simulink model "quadcopter_wind"  (Simulink 9.0)
settings: Solver=ode45  StartTime=0.0  StopTime=30  FixedStep=0.001  RelTol=1e-3  EnableMultiTasking=on
values from neighbouring files (symbols this model uses):
  C = 1    [control_params.m]
  f_phi = 10    [control_params.m]
  f_psi = 0.1    [control_params.m]
  f_theta = 0.1    [control_params.m]
  f_x = 10    [control_params.m]
  f_y = 10    [control_params.m]
  f_z = 10    [control_params.m]
  g = 9.8    [control_params.m]
  J_1 = 1    [control_params.m]
  J_2 = 1    [control_params.m]
  J_3 = 1    [control_params.m]
  l = 0.5    [control_params.m]
  m = 1    [control_params.m]
  phi_desired = 1    [control_params.m]
  x_desired = 1    [control_params.m]
  y_desired = 1    [control_params.m]
  z_desired = 1    [control_params.m]
settings Model: Creator=Oleg Borisov  LastModifiedBy=broth
settings DataIOCC: LimitDataPoints=on  SignalLoggingSaveFormat=ModelDataLogs
settings OptimizationCC: ExpressionDepthLimit=2147483647
settings DebuggingCC: SolverPrmCheckMsg=warning  FcnCallInpInsideContextMsg=warning  StateNameClashWarn=warning
settings GRTTargetCC: GeneratePreprocessorConditionals=Disable all  CombineOutputUpdateFcns=off  GRTInterface=on

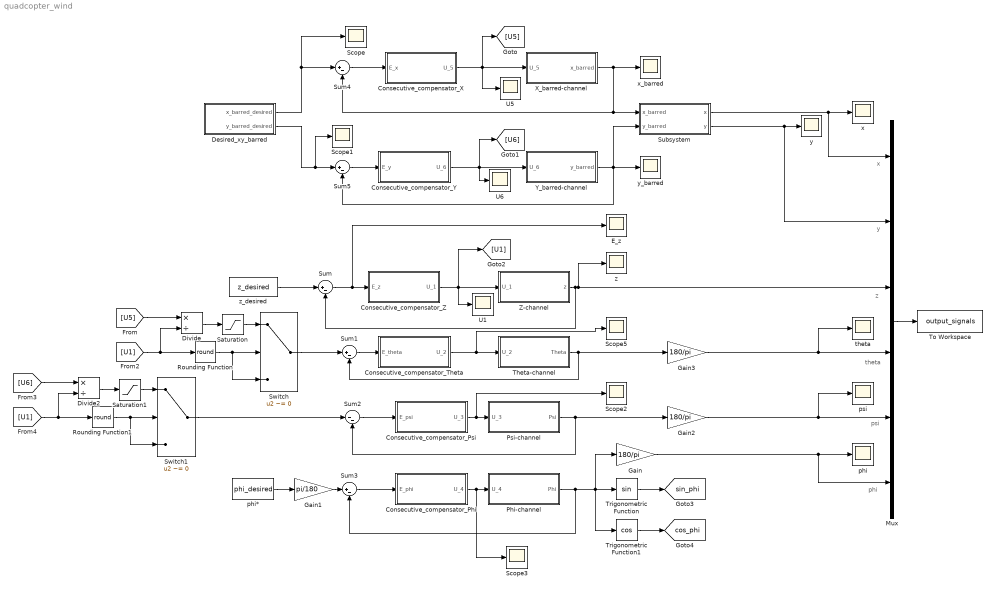
== system quadcopter_wind ==
  note: z
  note: y
  note: x
  note: theta
  note: psi
  note: phi
  Consecutive_compensator_Phi : Subsystem
  Consecutive_compensator_Psi : Subsystem
  Consecutive_compensator_Theta : Subsystem
  Consecutive_compensator_X : Subsystem
  Consecutive_compensator_Y : Subsystem
  Consecutive_compensator_Z : Subsystem
  Desired_xy_barred : Subsystem
  Divide : Product  Inputs=*/
  Divide2 : Product  Inputs=*/
  E_z : Scope
  Gain : Gain  Gain=180/pi
  Gain1 : Gain  Gain=pi/180
  Gain2 : Gain  Gain=180/pi
  Gain3 : Gain  Gain=180/pi
  Mux : Mux  Inputs=6
  Phi-channel : Subsystem
  Psi-channel : Subsystem
  Rounding Function : Rounding  Operator=round
  Rounding Function1 : Rounding  Operator=round
  Saturation : Saturate  UpperLimit=pi/6  LowerLimit=-pi/6
  Saturation1 : Saturate  UpperLimit=pi/6  LowerLimit=-pi/6
  Scope{,1..3,5} (5 alike) : Scope
  Subsystem : Subsystem
  Sum{,1,3..5} (5 alike) : Sum  Inputs=|+-
  Sum2 : Sum  Inputs=|--
  Switch : Switch  Criteria=u2 ~= 0
  Switch1 : Switch  Criteria=u2 ~= 0
  Theta-channel : Subsystem
  To Workspace : ToWorkspace  VariableName=output_signals  SaveFormat=Structure With Time  SampleTime=-1
  Trigonometric Function : Trigonometry
  Trigonometric Function1 : Trigonometry  Operator=cos
  U1 : Scope
  U5 : Scope
  U6 : Scope
  X_barred-channel : Subsystem
  Y_barred-channel : Subsystem
  Z-channel : Subsystem
  phi : Scope
  phi* : Constant  Value=phi_desired
  psi : Scope
  theta : Scope
  x : Scope
  x_barred : Scope
  y : Scope
  y_barred : Scope
  z : Scope
  z_desired : Constant  Value=z_desired
  tag scope: cos_phi=global, sin_phi=global
  wires:
  Z-channel/1(z) -> Mux/3, z/1, Sum/2
  Sum/1 -> E_z/1, Consecutive_compensator_Z/1(E_z)
  Consecutive_compensator_Psi/1(U_3) -> Psi-channel/1(U_3), Scope2/1
  Consecutive_compensator_Phi/1(U_4) -> Phi-channel/1(U_4), Scope3/1
  Theta-channel/1(Theta) -> Sum1/2, Gain3/1
  Sum1/1 -> Consecutive_compensator_Theta/1(E_theta)
  Sum2/1 -> Consecutive_compensator_Psi/1(E_psi)
  Psi-channel/1(Psi) -> Sum2/2, Gain2/1
  Sum3/1 -> Consecutive_compensator_Phi/1(E_phi)
  Phi-channel/1(Phi) -> Sum3/2, Trigonometric Function/1, Trigonometric Function1/1, Gain/1
  Consecutive_compensator_Y/1(U_6) -> Y_barred-channel/1(U_6), [U6], U6/1
  [U5] -> Divide/1
  X_barred-channel/1(x_barred) -> x_barred/1, Subsystem/1(x_barred), Sum4/2
  Sum5/1 -> Consecutive_compensator_Y/1(E_y)
  Y_barred-channel/1(y_barred) -> y_barred/1, Sum5/2, Subsystem/2(y_barred)
  Desired_xy_barred/1(x_barred_desired) -> Sum4/1, Scope/1
  Desired_xy_barred/2(y_barred_desired) -> Sum5/1, Scope1/1
  Trigonometric Function/1 -> [sin_phi]
  Trigonometric Function1/1 -> [cos_phi]
  Gain/1 -> Mux/6, phi/1
  phi*/1 -> Gain1/1
  Gain1/1 -> Sum3/1
  Mux/1 -> To Workspace/1
  Subsystem/1(x) -> Mux/1, x/1
  Subsystem/2(y) -> Mux/2, y/1
  Gain2/1 -> Mux/5, psi/1
  Gain3/1 -> Mux/4, theta/1
  Sum4/1 -> Consecutive_compensator_X/1(E_x)
  Consecutive_compensator_X/1(U_5) -> X_barred-channel/1(U_5), [U5], U5/1
  Consecutive_compensator_Z/1(U_1) -> Z-channel/1(U_1), [U1], U1/1
  z_desired/1 -> Sum/1
  Divide/1 -> Saturation/1
  [U1] -> Divide/2, Rounding Function/1
  Switch/1 -> Sum1/1
  Saturation/1 -> Switch/1
  Rounding Function/1 -> Switch/2, Switch/3
  Consecutive_compensator_Theta/1(U_2) -> Theta-channel/1(U_2), Scope5/1
  [U6] -> Divide2/1
  Divide2/1 -> Saturation1/1
  [U1] -> Divide2/2, Rounding Function1/1
  Saturation1/1 -> Switch1/1
  Rounding Function1/1 -> Switch1/2, Switch1/3
  Switch1/1 -> Sum2/1

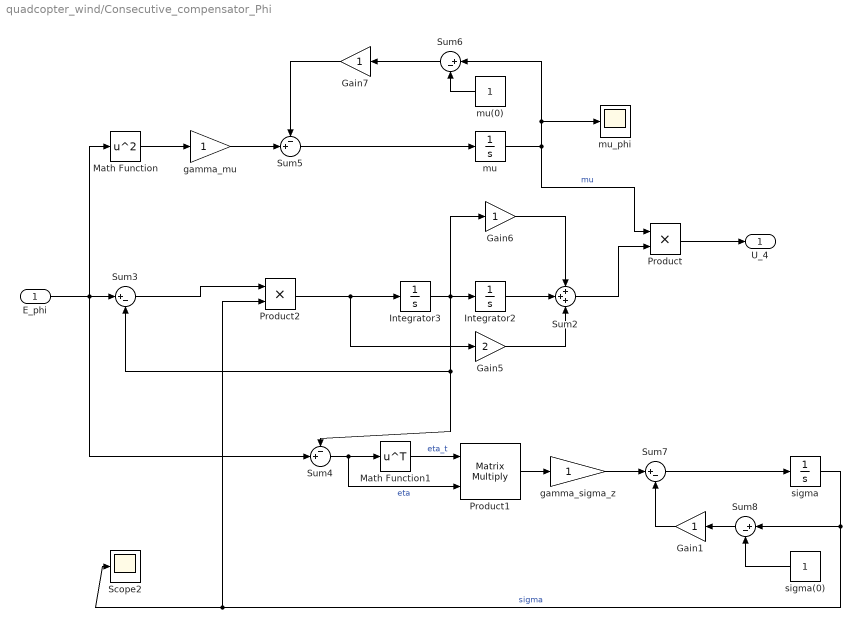
== system quadcopter_wind/Consecutive_compensator_Phi ==
  E_phi : Inport
  Gain1 : Gain
  Gain5 : Gain  Gain=2
  Gain6 : Gain
  Gain7 : Gain
  Integrator2 : Integrator
  Integrator3 : Integrator
  Math Function : Math  Operator=square  SaturateOnIntegerOverflow=on
  Math Function1 : Math  Operator=transpose  SaturateOnIntegerOverflow=on
  Product : Product
  Product1 : Product  Multiplication=Matrix(*)
  Product2 : Product
  Scope2 : Scope
  Sum2 : Sum  Inputs=+++
  Sum{3,6..8} (4 alike) : Sum  Inputs=|+-
  Sum4 : Sum  Inputs=-+|
  Sum5 : Sum  Inputs=-+|
  gamma_mu : Gain
  gamma_sigma_z : Gain
  mu : Integrator  InitialCondition=1
  mu(0) : Constant
  mu_phi : Scope
  sigma : Integrator  InitialCondition=1
  sigma(0) : Constant
  U_4 : Outport
  wires:
  Product2/1 -> Integrator3/1, Gain5/1
  Sum3/1 -> Product2/1
  Integrator2/1 -> Sum2/2
  Product/1 -> U_4/1
  Gain7/1 -> Sum5/1
  Sum2/1 -> Product/2
  mu/1 -> Product/1, mu_phi/1, Sum6/1  "mu"
  Gain6/1 -> Sum2/1
  mu(0)/1 -> Sum6/2
  Gain5/1 -> Sum2/3
  Sum5/1 -> mu/1
  Sum6/1 -> Gain7/1
  gamma_mu/1 -> Sum5/2
  Math Function/1 -> gamma_mu/1
  E_phi/1 -> Sum4/2, Math Function/1, Sum3/1
  Gain1/1 -> Sum7/2
  gamma_sigma_z/1 -> Sum7/1
  Sum7/1 -> sigma/1
  Sum8/1 -> Gain1/1
  sigma(0)/1 -> Sum8/2
  Sum4/1 -> Product1/2, Math Function1/1  "eta"
  Product1/1 -> gamma_sigma_z/1
  Integrator3/1 -> Integrator2/1, Gain6/1, Sum3/2, Sum4/1
  sigma/1 -> Sum8/1, Product2/2, Scope2/1  "sigma"
  Math Function1/1 -> Product1/1  "eta_t"

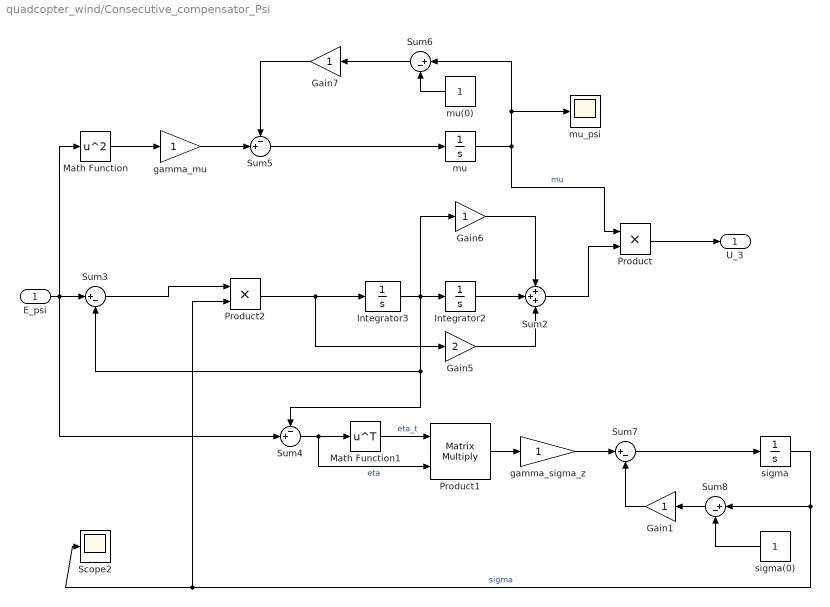
== system quadcopter_wind/Consecutive_compensator_Psi ==
  E_psi : Inport
  Gain1 : Gain
  Gain5 : Gain  Gain=2
  Gain6 : Gain
  Gain7 : Gain
  Integrator2 : Integrator
  Integrator3 : Integrator
  Math Function : Math  Operator=square  SaturateOnIntegerOverflow=on
  Math Function1 : Math  Operator=transpose  SaturateOnIntegerOverflow=on
  Product : Product
  Product1 : Product  Multiplication=Matrix(*)
  Product2 : Product
  Scope2 : Scope
  Sum2 : Sum  Inputs=+++
  Sum{3,6..8} (4 alike) : Sum  Inputs=|+-
  Sum4 : Sum  Inputs=-+|
  Sum5 : Sum  Inputs=-+|
  gamma_mu : Gain
  gamma_sigma_z : Gain
  mu : Integrator  InitialCondition=1
  mu(0) : Constant
  mu_psi : Scope
  sigma : Integrator  InitialCondition=1
  sigma(0) : Constant
  U_3 : Outport
  wires:
  Product2/1 -> Integrator3/1, Gain5/1
  Sum3/1 -> Product2/1
  Integrator2/1 -> Sum2/2
  Product/1 -> U_3/1
  Gain7/1 -> Sum5/1
  Sum2/1 -> Product/2
  mu/1 -> Product/1, mu_psi/1, Sum6/1  "mu"
  Gain6/1 -> Sum2/1
  mu(0)/1 -> Sum6/2
  Gain5/1 -> Sum2/3
  Sum5/1 -> mu/1
  Sum6/1 -> Gain7/1
  gamma_mu/1 -> Sum5/2
  Math Function/1 -> gamma_mu/1
  E_psi/1 -> Math Function/1, Sum4/2, Sum3/1
  Gain1/1 -> Sum7/2
  gamma_sigma_z/1 -> Sum7/1
  Sum7/1 -> sigma/1
  Sum8/1 -> Gain1/1
  sigma(0)/1 -> Sum8/2
  Sum4/1 -> Product1/2, Math Function1/1  "eta"
  Product1/1 -> gamma_sigma_z/1
  Integrator3/1 -> Integrator2/1, Gain6/1, Sum4/1, Sum3/2
  sigma/1 -> Sum8/1, Product2/2, Scope2/1  "sigma"
  Math Function1/1 -> Product1/1  "eta_t"

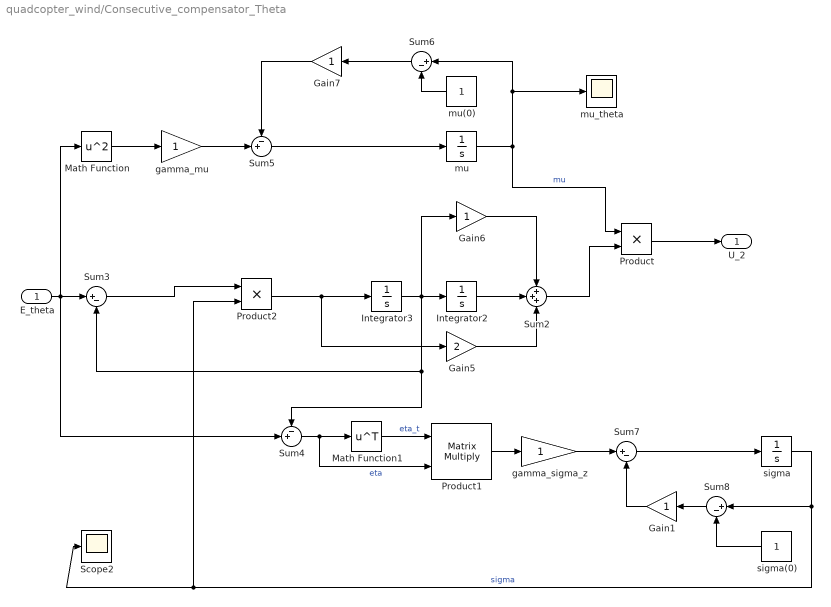
== system quadcopter_wind/Consecutive_compensator_Theta ==
  E_theta : Inport
  Gain1 : Gain
  Gain5 : Gain  Gain=2
  Gain6 : Gain
  Gain7 : Gain
  Integrator2 : Integrator
  Integrator3 : Integrator
  Math Function : Math  Operator=square  SaturateOnIntegerOverflow=on
  Math Function1 : Math  Operator=transpose  SaturateOnIntegerOverflow=on
  Product : Product
  Product1 : Product  Multiplication=Matrix(*)
  Product2 : Product
  Scope2 : Scope
  Sum2 : Sum  Inputs=+++
  Sum{3,6..8} (4 alike) : Sum  Inputs=|+-
  Sum4 : Sum  Inputs=-+|
  Sum5 : Sum  Inputs=-+|
  gamma_mu : Gain
  gamma_sigma_z : Gain
  mu : Integrator  InitialCondition=1
  mu(0) : Constant
  mu_theta : Scope
  sigma : Integrator  InitialCondition=1
  sigma(0) : Constant
  U_2 : Outport
  wires:
  Product2/1 -> Integrator3/1, Gain5/1
  Sum3/1 -> Product2/1
  Integrator2/1 -> Sum2/2
  Product/1 -> U_2/1
  Gain7/1 -> Sum5/1
  Sum2/1 -> Product/2
  mu/1 -> Product/1, mu_theta/1, Sum6/1  "mu"
  Gain6/1 -> Sum2/1
  mu(0)/1 -> Sum6/2
  Gain5/1 -> Sum2/3
  Sum5/1 -> mu/1
  Sum6/1 -> Gain7/1
  gamma_mu/1 -> Sum5/2
  Math Function/1 -> gamma_mu/1
  E_theta/1 -> Sum4/2, Math Function/1, Sum3/1
  Gain1/1 -> Sum7/2
  gamma_sigma_z/1 -> Sum7/1
  Sum7/1 -> sigma/1
  Sum8/1 -> Gain1/1
  sigma(0)/1 -> Sum8/2
  Sum4/1 -> Product1/2, Math Function1/1  "eta"
  Product1/1 -> gamma_sigma_z/1
  Integrator3/1 -> Integrator2/1, Gain6/1, Sum3/2, Sum4/1
  sigma/1 -> Sum8/1, Product2/2, Scope2/1  "sigma"
  Math Function1/1 -> Product1/1  "eta_t"

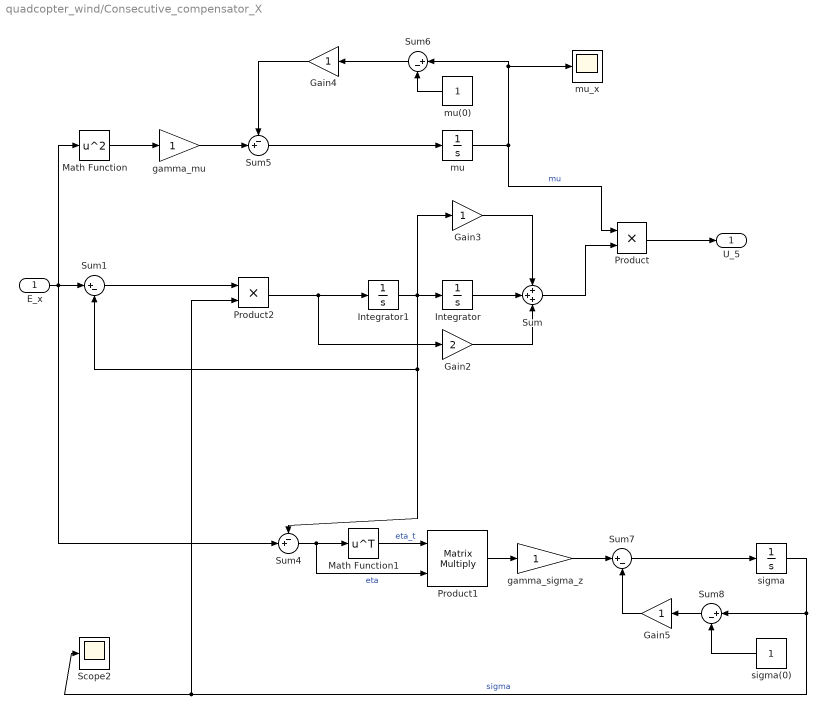
== system quadcopter_wind/Consecutive_compensator_X ==
  E_x : Inport
  Gain2 : Gain  Gain=2
  Gain3 : Gain
  Gain4 : Gain
  Gain5 : Gain
  Integrator : Integrator
  Integrator1 : Integrator
  Math Function : Math  Operator=square  SaturateOnIntegerOverflow=on
  Math Function1 : Math  Operator=transpose  SaturateOnIntegerOverflow=on
  Product : Product
  Product1 : Product  Multiplication=Matrix(*)
  Product2 : Product
  Scope2 : Scope
  Sum : Sum  Inputs=+++
  Sum{1,6..8} (4 alike) : Sum  Inputs=|+-
  Sum4 : Sum  Inputs=-+|
  Sum5 : Sum  Inputs=-+|
  gamma_mu : Gain
  gamma_sigma_z : Gain
  mu : Integrator  InitialCondition=1
  mu(0) : Constant
  mu_x : Scope
  sigma : Integrator  InitialCondition=1
  sigma(0) : Constant
  U_5 : Outport
  wires:
  Sum/1 -> Product/2
  Integrator/1 -> Sum/2
  Sum1/1 -> Product2/1
  Product2/1 -> Integrator1/1, Gain2/1
  Gain3/1 -> Sum/1
  Gain2/1 -> Sum/3
  gamma_mu/1 -> Sum5/2
  mu(0)/1 -> Sum6/2
  Sum6/1 -> Gain4/1
  Math Function/1 -> gamma_mu/1
  mu/1 -> Product/1, mu_x/1, Sum6/1  "mu"
  Gain4/1 -> Sum5/1
  Sum5/1 -> mu/1
  Product/1 -> U_5/1
  sigma(0)/1 -> Sum8/2
  sigma/1 -> Sum8/1, Product2/2, Scope2/1  "sigma"
  Sum8/1 -> Gain5/1
  Math Function1/1 -> Product1/1  "eta_t"
  Gain5/1 -> Sum7/2
  gamma_sigma_z/1 -> Sum7/1
  E_x/1 -> Sum4/2, Math Function/1, Sum1/1
  Integrator1/1 -> Integrator/1, Gain3/1, Sum4/1, Sum1/2
  Sum7/1 -> sigma/1
  Sum4/1 -> Product1/2, Math Function1/1  "eta"
  Product1/1 -> gamma_sigma_z/1

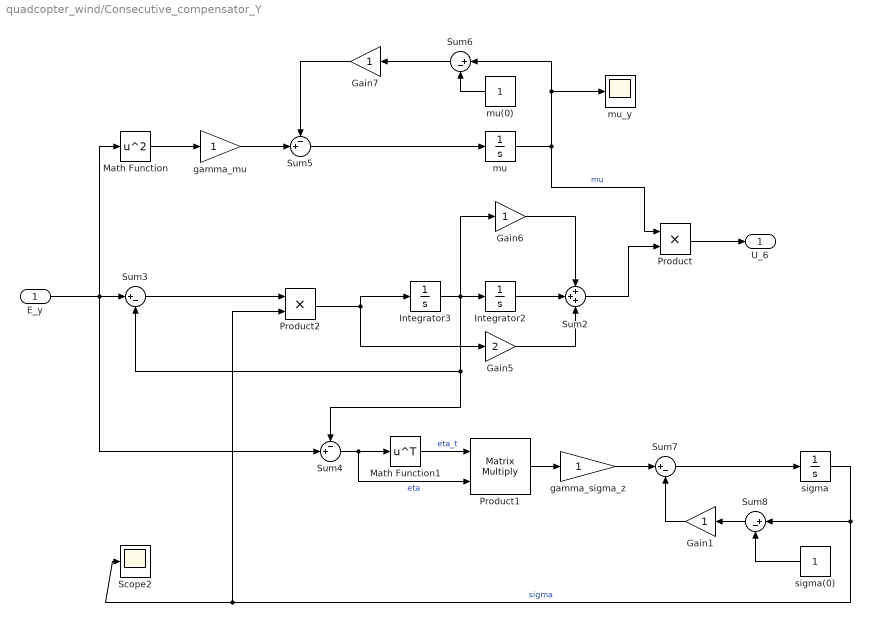
== system quadcopter_wind/Consecutive_compensator_Y ==
  E_y : Inport
  Gain1 : Gain
  Gain5 : Gain  Gain=2
  Gain6 : Gain
  Gain7 : Gain
  Integrator2 : Integrator
  Integrator3 : Integrator
  Math Function : Math  Operator=square  SaturateOnIntegerOverflow=on
  Math Function1 : Math  Operator=transpose  SaturateOnIntegerOverflow=on
  Product : Product
  Product1 : Product  Multiplication=Matrix(*)
  Product2 : Product
  Scope2 : Scope
  Sum2 : Sum  Inputs=+++
  Sum{3,6..8} (4 alike) : Sum  Inputs=|+-
  Sum4 : Sum  Inputs=-+|
  Sum5 : Sum  Inputs=-+|
  gamma_mu : Gain
  gamma_sigma_z : Gain
  mu : Integrator  InitialCondition=1
  mu(0) : Constant
  mu_y : Scope
  sigma : Integrator  InitialCondition=1
  sigma(0) : Constant
  U_6 : Outport
  wires:
  Product/1 -> U_6/1
  Product2/1 -> Integrator3/1, Gain5/1
  Sum3/1 -> Product2/1
  Integrator2/1 -> Sum2/2
  Gain7/1 -> Sum5/1
  Sum2/1 -> Product/2
  mu/1 -> Product/1, mu_y/1, Sum6/1  "mu"
  Gain6/1 -> Sum2/1
  mu(0)/1 -> Sum6/2
  Gain5/1 -> Sum2/3
  Sum5/1 -> mu/1
  Sum6/1 -> Gain7/1
  gamma_mu/1 -> Sum5/2
  Math Function/1 -> gamma_mu/1
  Integrator3/1 -> Integrator2/1, Gain6/1, Sum3/2, Sum4/1
  Sum7/1 -> sigma/1
  gamma_sigma_z/1 -> Sum7/1
  Gain1/1 -> Sum7/2
  Sum4/1 -> Product1/2, Math Function1/1  "eta"
  Sum8/1 -> Gain1/1
  sigma(0)/1 -> Sum8/2
  Product1/1 -> gamma_sigma_z/1
  Math Function1/1 -> Product1/1  "eta_t"
  sigma/1 -> Sum8/1, Product2/2, Scope2/1  "sigma"
  E_y/1 -> Sum3/1, Sum4/2, Math Function/1

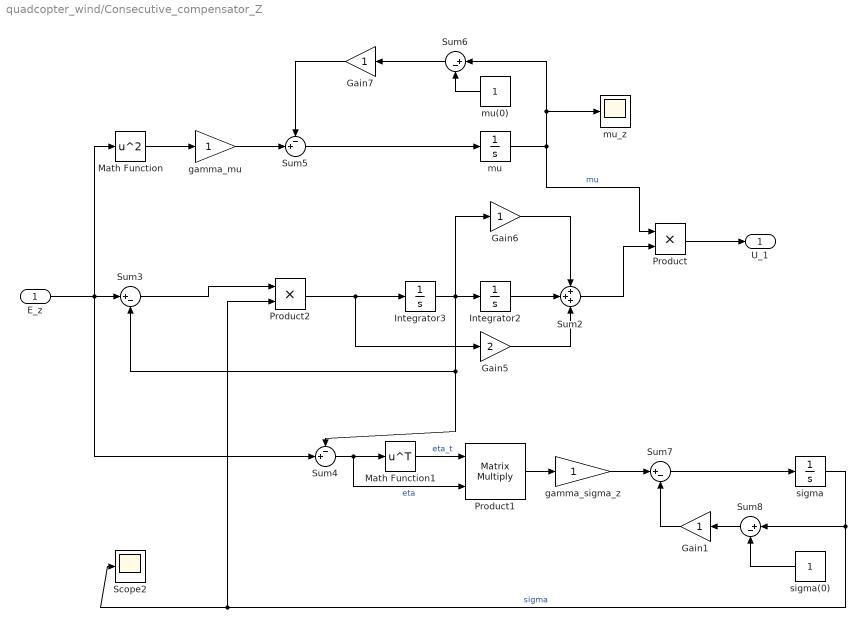
== system quadcopter_wind/Consecutive_compensator_Z ==
  E_z : Inport
  Gain1 : Gain
  Gain5 : Gain  Gain=2
  Gain6 : Gain
  Gain7 : Gain
  Integrator2 : Integrator
  Integrator3 : Integrator
  Math Function : Math  Operator=square  SaturateOnIntegerOverflow=on
  Math Function1 : Math  Operator=transpose  SaturateOnIntegerOverflow=on
  Product : Product
  Product1 : Product  Multiplication=Matrix(*)
  Product2 : Product
  Scope2 : Scope
  Sum2 : Sum  Inputs=+++
  Sum{3,6..8} (4 alike) : Sum  Inputs=|+-
  Sum4 : Sum  Inputs=-+|
  Sum5 : Sum  Inputs=-+|
  gamma_mu : Gain
  gamma_sigma_z : Gain
  mu : Integrator  InitialCondition=1
  mu(0) : Constant
  mu_z : Scope
  sigma : Integrator  InitialCondition=1
  sigma(0) : Constant
  U_1 : Outport
  wires:
  Product/1 -> U_1/1
  Product2/1 -> Integrator3/1, Gain5/1
  Sum3/1 -> Product2/1
  Integrator2/1 -> Sum2/2
  Gain7/1 -> Sum5/1
  Sum2/1 -> Product/2
  mu/1 -> Product/1, mu_z/1, Sum6/1  "mu"
  Gain6/1 -> Sum2/1
  mu(0)/1 -> Sum6/2
  Gain5/1 -> Sum2/3
  Sum5/1 -> mu/1
  Sum6/1 -> Gain7/1
  gamma_mu/1 -> Sum5/2
  Math Function/1 -> gamma_mu/1
  Math Function1/1 -> Product1/1  "eta_t"
  E_z/1 -> Sum4/2, Math Function/1, Sum3/1
  sigma/1 -> Sum8/1, Product2/2, Scope2/1  "sigma"
  Sum4/1 -> Product1/2, Math Function1/1  "eta"
  Product1/1 -> gamma_sigma_z/1
  gamma_sigma_z/1 -> Sum7/1
  Sum8/1 -> Gain1/1
  sigma(0)/1 -> Sum8/2
  Sum7/1 -> sigma/1
  Integrator3/1 -> Integrator2/1, Gain6/1, Sum3/2, Sum4/1
  Gain1/1 -> Sum7/2

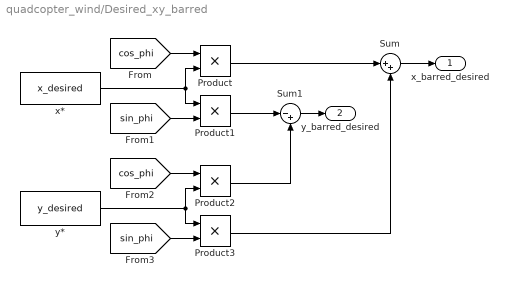
== system quadcopter_wind/Desired_xy_barred ==
  Product{,1..3} (4 alike) : Product  RndMeth=Zero
  Sum : Sum  Inputs=|++
  Sum1 : Sum  Inputs=|-+
  x* : Constant  Value=x_desired
  y* : Constant  Value=y_desired
  x_barred_desired : Outport
  y_barred_desired : Outport  Port=2
  wires:
  [cos_phi] -> Product/1
  [sin_phi] -> Product1/2
  [cos_phi] -> Product2/1
  [sin_phi] -> Product3/2
  Product/1 -> Sum/1
  Product3/1 -> Sum/2
  Product1/1 -> Sum1/1
  Product2/1 -> Sum1/2
  Sum/1 -> x_barred_desired/1
  Sum1/1 -> y_barred_desired/1
  x*/1 -> Product/2, Product1/1
  y*/1 -> Product2/2, Product3/1

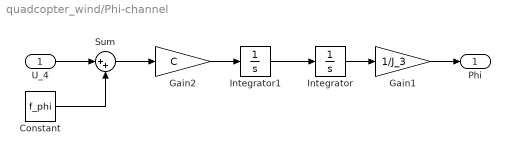
== system quadcopter_wind/Phi-channel ==
  U_4 : Inport
  Constant : Constant  Value=f_phi
  Gain1 : Gain  Gain=1/J_3
  Gain2 : Gain  Gain=C
  Integrator : Integrator
  Integrator1 : Integrator
  Sum : Sum  Inputs=|++
  Phi : Outport
  wires:
  Integrator1/1 -> Integrator/1
  Integrator/1 -> Gain1/1
  Gain1/1 -> Phi/1
  Gain2/1 -> Integrator1/1
  U_4/1 -> Sum/1
  Sum/1 -> Gain2/1
  Constant/1 -> Sum/2

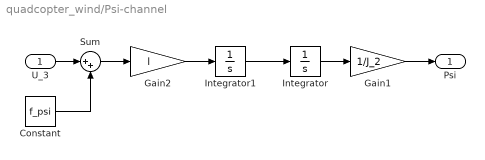
== system quadcopter_wind/Psi-channel ==
  U_3 : Inport
  Constant : Constant  Value=f_psi
  Gain1 : Gain  Gain=1/J_2
  Gain2 : Gain  Gain=l
  Integrator : Integrator
  Integrator1 : Integrator
  Sum : Sum  Inputs=|++
  Psi : Outport
  wires:
  Integrator1/1 -> Integrator/1
  Integrator/1 -> Gain1/1
  Gain1/1 -> Psi/1
  Gain2/1 -> Integrator1/1
  U_3/1 -> Sum/1
  Sum/1 -> Gain2/1
  Constant/1 -> Sum/2

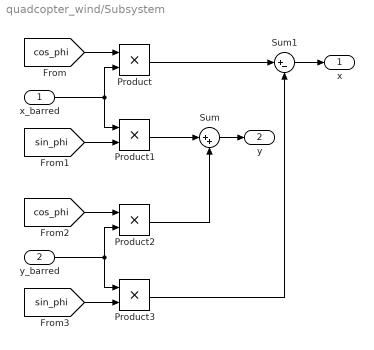
== system quadcopter_wind/Subsystem ==
  x_barred : Inport
  y_barred : Inport  Port=2
  Product{,1..3} (4 alike) : Product  RndMeth=Zero
  Sum : Sum  Inputs=|++
  Sum1 : Sum  Inputs=|+-
  x : Outport
  y : Outport  Port=2
  wires:
  [cos_phi] -> Product/1
  [sin_phi] -> Product1/2
  x_barred/1 -> Product/2, Product1/1
  [cos_phi] -> Product2/1
  [sin_phi] -> Product3/2
  y_barred/1 -> Product2/2, Product3/1
  Product1/1 -> Sum/1
  Product2/1 -> Sum/2
  Product/1 -> Sum1/1
  Product3/1 -> Sum1/2
  Sum1/1 -> x/1
  Sum/1 -> y/1

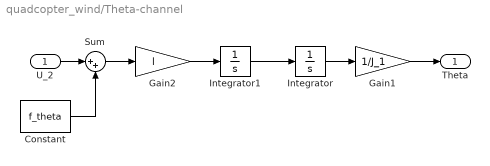
== system quadcopter_wind/Theta-channel ==
  U_2 : Inport
  Constant : Constant  Value=f_theta
  Gain1 : Gain  Gain=1/J_1
  Gain2 : Gain  Gain=l
  Integrator : Integrator
  Integrator1 : Integrator
  Sum : Sum  Inputs=|++
  Theta : Outport
  wires:
  Integrator1/1 -> Integrator/1
  Integrator/1 -> Gain1/1
  Gain1/1 -> Theta/1
  Gain2/1 -> Integrator1/1
  U_2/1 -> Sum/1
  Sum/1 -> Gain2/1
  Constant/1 -> Sum/2

== system quadcopter_wind/X_barred-channel ==
  U_5 : Inport
  Constant : Constant  Value=f_x
  Gain1 : Gain  Gain=1/m
  Integrator : Integrator
  Integrator1 : Integrator
  Sum : Sum  Inputs=|++
  x_barred : Outport
  wires:
  Integrator1/1 -> Integrator/1
  Integrator/1 -> Gain1/1
  Gain1/1 -> x_barred/1
  U_5/1 -> Sum/1
  Sum/1 -> Integrator1/1
  Constant/1 -> Sum/2

== system quadcopter_wind/Y_barred-channel ==
  U_6 : Inport
  Constant : Constant  Value=f_y
  Gain1 : Gain  Gain=1/m
  Integrator : Integrator
  Integrator1 : Integrator
  Sum : Sum  Inputs=|++
  y_barred : Outport
  wires:
  Integrator1/1 -> Integrator/1
  Integrator/1 -> Gain1/1
  Gain1/1 -> y_barred/1
  U_6/1 -> Sum/1
  Sum/1 -> Integrator1/1
  Constant/1 -> Sum/2

== system quadcopter_wind/Z-channel ==
  U_1 : Inport
  Constant : Constant  Value=m*g
  Constant1 : Constant  Value=f_z
  Gain1 : Gain  Gain=1/m
  Integrator : Integrator
  Integrator1 : Integrator
  Sum : Sum  Inputs=++-
  z : Outport
  wires:
  Sum/1 -> Integrator1/1
  Integrator1/1 -> Integrator/1
  Integrator/1 -> Gain1/1
  Gain1/1 -> z/1
  Constant/1 -> Sum/3
  U_1/1 -> Sum/2
  Constant1/1 -> Sum/1
